simulink model "empty"  (R2021a)
settings: Solver=VariableStepAuto  StartTime=0.0  StopTime=10.0  RelTol=1e-3
settings Model: Creator=quratulainali  LastModifiedBy=quratulainali

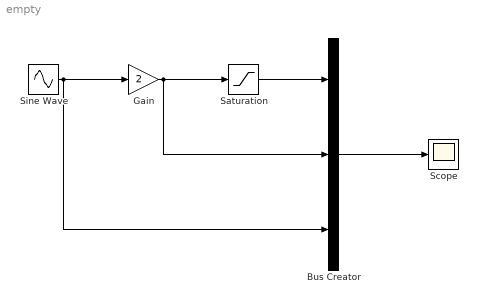
== system empty ==
  Bus Creator : BusCreator  Inputs=3
  Gain : Gain  Gain=2
  Saturation : Saturate
  Scope : Scope
  Sine Wave : Sin  SampleTime=0
  wires:
  Sine Wave/1 -> Gain/1, Bus Creator/3
  Gain/1 -> Saturation/1, Bus Creator/2
  Saturation/1 -> Bus Creator/1
  Bus Creator/1 -> Scope/1
